simulink library "INT_CrC_VD"  (R2016b)
settings: Solver=VariableStepAuto  StartTime=0.0  StopTime=10.0  RelTol=1e-3
settings Model: Creator=xinchangran  LastModifiedBy=xinchangran

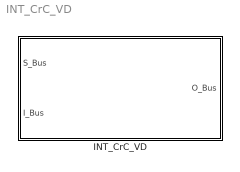
== system INT_CrC_VD ==
  INT_CrC_VD : Subsystem

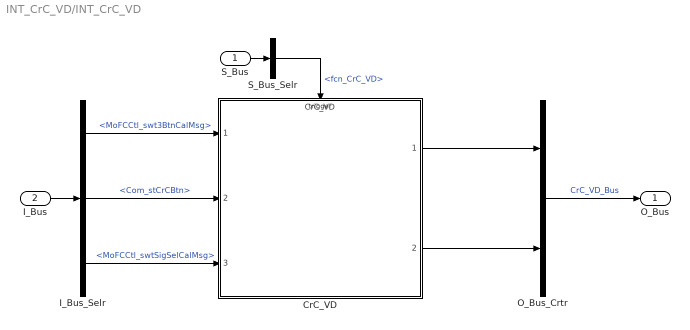
== system INT_CrC_VD/INT_CrC_VD ==
  S_Bus : Inport
  I_Bus : Inport  Port=2
  CrC_VD : ModelReference  ModelNameDialog=CrC_VD  SimulationMode=Normal  ModelReferenceVersion=1.50  TriggerPortName=function  TriggerPortTriggerType=function-call  TriggerPortStatesWhenEnabling=held
  I_Bus_Selr : BusSelector  OutputSignals=MoFCCtl_swt3BtnCalMsg,Com_stCrCBtn,MoFCCtl_swtSigSelCalMsg
  O_Bus_Crtr : BusCreator  Inputs=2
  S_Bus_Selr : BusSelector  OutputSignals=fcn_CrC_VD
  O_Bus : Outport
  wires:
  S_Bus_Selr/1 -> CrC_VD/Trigger  "<fcn_CrC_VD>"
  S_Bus/1 -> S_Bus_Selr/1
  I_Bus/1 -> I_Bus_Selr/1
  I_Bus_Selr/1 -> CrC_VD/1  "<MoFCCtl_swt3BtnCalMsg>"
  I_Bus_Selr/2 -> CrC_VD/2  "<Com_stCrCBtn>"
  I_Bus_Selr/3 -> CrC_VD/3  "<MoFCCtl_swtSigSelCalMsg>"
  O_Bus_Crtr/1 -> O_Bus/1  "CrC_VD_Bus"
  CrC_VD/1 -> O_Bus_Crtr/1
  CrC_VD/2 -> O_Bus_Crtr/2
